simulink model "transfer_function_test"  (R2023a)
settings: Solver=VariableStepAuto  StartTime=0.0  StopTime=1  RelTol=1e-3
values from neighbouring files (symbols this model uses):
  h = 10e-3    (= 0.01)    [tranf_func_test.m]
  Kt = 1e-3    (= 0.001)    [tranf_func_test.m]
libraries: cstblocks x2
settings Model: Creator=under  LastModifiedBy=under

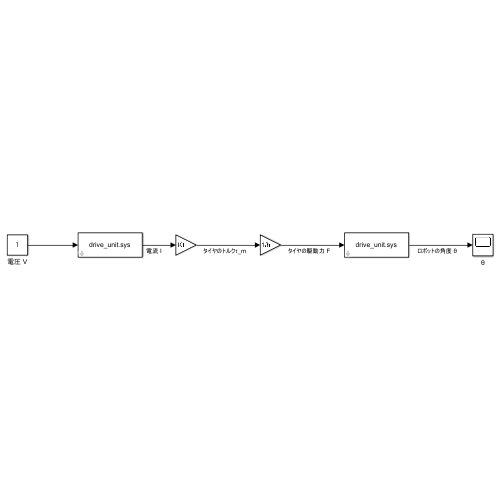
[thumbnail: Simulink's stored preview of the top-level diagram]
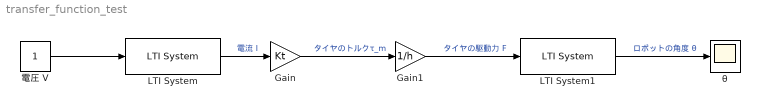
== system transfer_function_test ==
  Gain : Gain  Gain=Kt
  Gain1 : Gain  Gain=1/h
  LTI System : cstblocks/LTI System  sys=drive_unit.sys  IC=[]
  LTI System1 : cstblocks/LTI System  sys=drive_unit.sys  IC=[]
  θ : Scope
  電圧 V : Constant
  wires:
  Gain1/1 -> LTI System1/1  "タイヤの駆動力 F"
  Gain/1 -> Gain1/1  "タイヤのトルクτ_m"
  LTI System/1 -> Gain/1  "電流 I"
  電圧 V/1 -> LTI System/1
  LTI System1/1 -> θ/1  "ロボットの角度 θ"
